simulink model "EOM_planar_vehicle_linmod"  (R2026a)
settings: Solver=VariableStepAuto  StopTime=10  MaxStep=deltaTMax
values from neighbouring files (symbols this model uses):
  CR = 0.75    [LineariseScript.m]    (also in PlanarVehicleScript.m)
  CT = 1/40    (= 0.025)    [LineariseScript.m]    (also in PlanarVehicleScript.m)
  Fmax = 10    [LineariseScript.m]    (also in PlanarVehicleScript.m)
  Ib = 0.5    [LineariseScript.m]    (also in PlanarVehicleScript.m)
  m = 10    [LineariseScript.m]    (also in PlanarVehicleScript.m)
  Mmax = 0.5    [LineariseScript.m]    (also in PlanarVehicleScript.m)
  u0 = [0.25 ... (first row only)    [LineariseScript.m]
  x0 = [10; -10; 0; 10; pi/2; 0]    [LineariseScript.m]    (also in PlanarVehicleScript.m = [10; -10; 0; 15; pi/2; 0])
settings Model: Creator=nuris  LastModifiedBy=nuris
settings DataIOCC: ExternalInput=getinputstruct(op_trim1)  InitialState=getstatestruct(op_trim1)

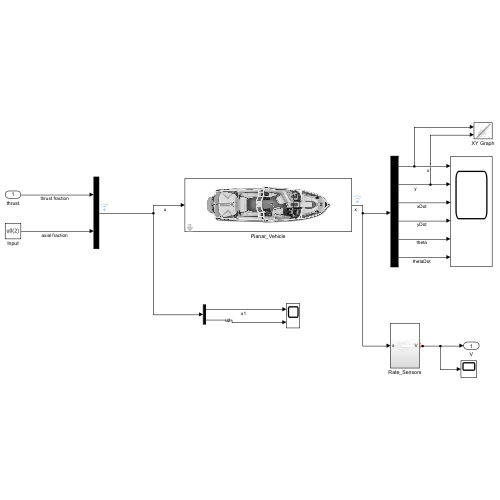
[thumbnail: Simulink's stored preview of the top-level diagram]
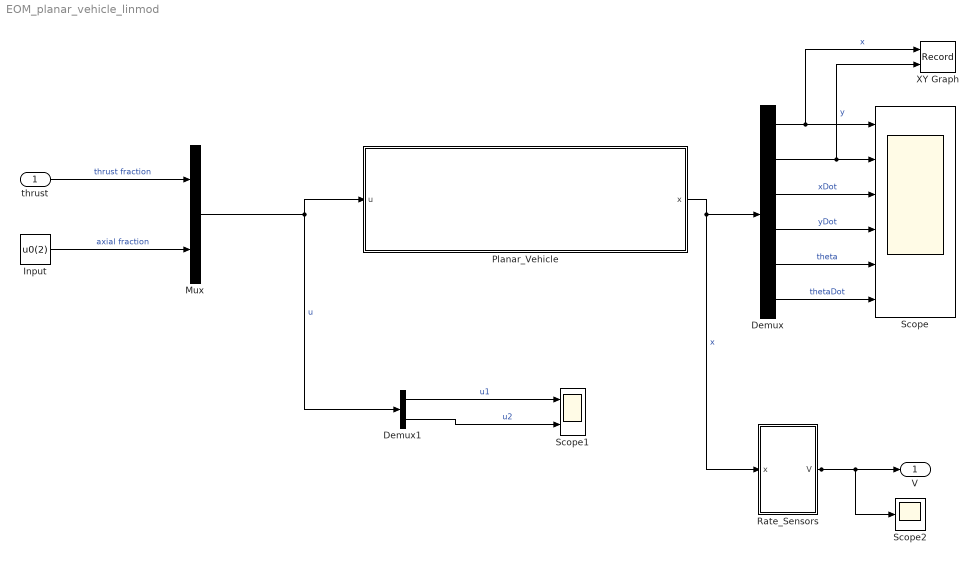
== system EOM_planar_vehicle_linmod ==
  thrust : Inport
  Demux : Demux  Outputs=6
  Demux1 : Demux  Outputs=2
  Input : Constant  Value=u0(2)
  Mux : Mux  Inputs=2
  Planar_Vehicle : Subsystem  mask(Subsystem (mask) (link)){x0=x0}
      mask prompts: x0 "Initial condition"
      mask help:
      | Represent a simple planar model.
      |
      | The state vector is
      |   x = [x;y;xdot;ydot;theta;thetadot]
      |
      | The control vector is
      |   u = [u1; u2]
      |
      | where:
      | u1 = fraction of axial thrust force in range [-1, 1] (-1 = full negative force, +1 = full positive force)
      | u2 = fraction of moment about CG in range [-1, 1] (-1 = full negative moment, +1 = full positive moment)
      |
      | INPUTS:
      |   u: 2x1 control vector
      |
      | OUTPUTS:
      |   x: 6x1 state vector
      mask Display: image(imread('C:\Users\nuris\Desktop\Michigan\Control\EOM_Planar_Vehicle\Boat.png'))
  Rate_Sensors : Subsystem
  Scope : Scope  NumInputPorts=6
      settings: ActiveDisplayYMinimum=-25.922686555926731  ActiveDisplayYMaximum=133.30417900334061
  Scope1 : Scope  NumInputPorts=2
      settings: ActiveDisplayYMinimum=-1  ActiveDisplayYMaximum=1
  Scope2 : Scope
      settings: ActiveDisplayYMinimum=14.999999999999581  ActiveDisplayYMaximum=15.000000000003784  DataLoggingVariableName=ScopeData2
  XY Graph : Record  NumPorts=2.0  FileSettingsInternal="{\"entries\":[{\"content\":{\"excelSettings\":{\"content\":{},\"type\":\"Streamout.ExcelSettings\"},\"parquetSettings\":{\"content\":{},\"type\":\"Streamout.ParquetSettings\"}},\"type\":\"Streamout.FileSettingStorage\",\"uuid\":\"\"}],\"packageUris\":[\"http:\\/\\/schema.mathworks.com\\/mf0\\/streamout_blocks\\/R2020a\"],\"version\":\"1.0\"}"  FrameSettings=[0, 0]  Layout=[1 1]  SignalsInternal="{\"entries\":[{\"content\":{\"signals\":[{\"content\":{\"blockPath\":[],\"dimensions\":[1],\"domain\":\"\",\"lineColor\":\"#edb120\",\"lineWidth\":2,\"port\":1,\"sid\":[\"\"],\"signalID\":1,\"signalName\":\"yDot\"},\"type\":\"RecordBlkView.Signal\",\"uuid\":\"\"},{\"content\":{\"blockPath\":[],\"dimensions\":[1],\"domain\":\"\",\"lineColor\":\"#7e2f8e\",\"lineWidth\":2,\"port\":1,\"sid\":[\"\"],\"signalID\":2},\"type\":\"RecordBlkView.Signal\",\"uuid\":\"\"},{\"content\":{\"blockPath\":[],\"dimensions\":[6],\"domain\":\"\",\"hasChildren\":true,\"lineColor\":\"#fe330a\",\"lineWidth\":2,\"port\":1,\"sid\":[\"\"],\"signalID\":3,\"signalName\":\"x\"},\"type\":\"RecordBlkView.Signal\",\"uuid\":\"\"},{\"content\":{\"blockPath\":[],\"channel\":[1],\"dimensions\":[6],\"domain\":\"\",\"lineColor\":\"#4dbeee\",\"lineWidth\":2,\"parentID\":3,\"port\":1,\"sid\":[\"\"],\"signalID\":4,\"signalName\":\"x\"},\"type\":\"RecordBlkView.Signal\",\"uuid\":\"\"},{\"content\":{\"blockPath\":[],\"dimensions\":[1],\"domain\":\"\",\"lineColor\":\"#a2142f\",\"plots\":[ 1 ],\"port\":1,\"sid\":[\"\"],\"signalID\":5,\"signalName\":\"x\"},\"type\":\"RecordBlkView.Signal\",\"uuid\":\"\"},{\"content\":{\"blockPath\":[],\"dimensions\":[1],\"domain\":\"\",\"lineColor\":\"#139fff\",\"plots\":[ 1 ],\"port\":2,\"sid\":[\"\"],\"signalID\":6,\"signalName\":\"y\"},\"type\":\"RecordBlkView.Signal\",\"uuid\":\"\"},{\"content\":{\"blockPath\":[],\"dimensions\":[2],\"domain\":\"\",\"hasChildren\":true,\"lineColor\":\"#edb120\",\"lineWidth\":2,\"port\":1,\"sid\":[\"\"],\"signalID\":7,\"signalName\":\"u\"},\"type\":\"RecordBlkView.Signal\",\"uuid\":\"\"},{\"content\":{\"blockPath\":[],\"channel\":[1],\"dimensions\":[2],\"domain\":\"\",\"lineColor\":\"#b746ff\",\"lineWidth\":2,\"parentID\":7,\"port\":1,\"sid\":[\"\"],\"signalID\":8,\"signalName\":\"u\"},\"type\":\"RecordBlkView.Signal\",\"uuid\":\"\"},{\"content\":{\"blockPath\":[],\"channel\":[2],\"dimensions\":[2],\"domain\":\"\",\"lineColor\":\"#77ac30\",\"lineWidth\":2,\"parentID\":7,\"port\":1,\"sid\":[\"\"],\"signalID\":9,\"signalName\":\"u\"},\"type\":\"RecordBlkView.Signal\",\"uuid\":\"\"}]},\"type\":\"RecordBlkView.InputSignals\",\"uuid\":\"\"}],\"packageUris\":[\"http:\\/\\/schema.mathworks.com\\/mf0\\/streamout_blocks\\/R2020a\"],\"version\":\"1.0\"}"  VisualizationBindings="{\"xyplotplugin\":{\"info\":[{\"series\":[{\"bindingParametersList\":[{\"parameter\":\"X-Axis\",\"signalID\":5,\"signalName\":\"x\"},{\"parameter\":\"Y-Axis\",\"signalID\":6,\"signalName\":\"y\"}],\"seriesID\":0}],\"subplotID\":1}]}}"  CompatibilityTag=XY
  V : Outport
  wires:
  Planar_Vehicle/1(x) -> Rate_Sensors/1(x), Demux/1  "x"
  Demux/1 -> XY Graph/1, Scope/1  "x"
  Demux/2 -> XY Graph/2, Scope/2  "y"
  Demux/3 -> Scope/3  "xDot"
  Demux/4 -> Scope/4  "yDot"
  Demux/5 -> Scope/5  "theta"
  Demux/6 -> Scope/6  "thetaDot"
  thrust/1 -> Mux/1  "thrust fraction"
  Input/1 -> Mux/2  "axial fraction"
  Mux/1 -> Demux1/1, Planar_Vehicle/1(u)  "u"
  Demux1/1 -> Scope1/1  "u1"
  Demux1/2 -> Scope1/2  "u2"
  Rate_Sensors/1(V) -> V/1, Scope2/1

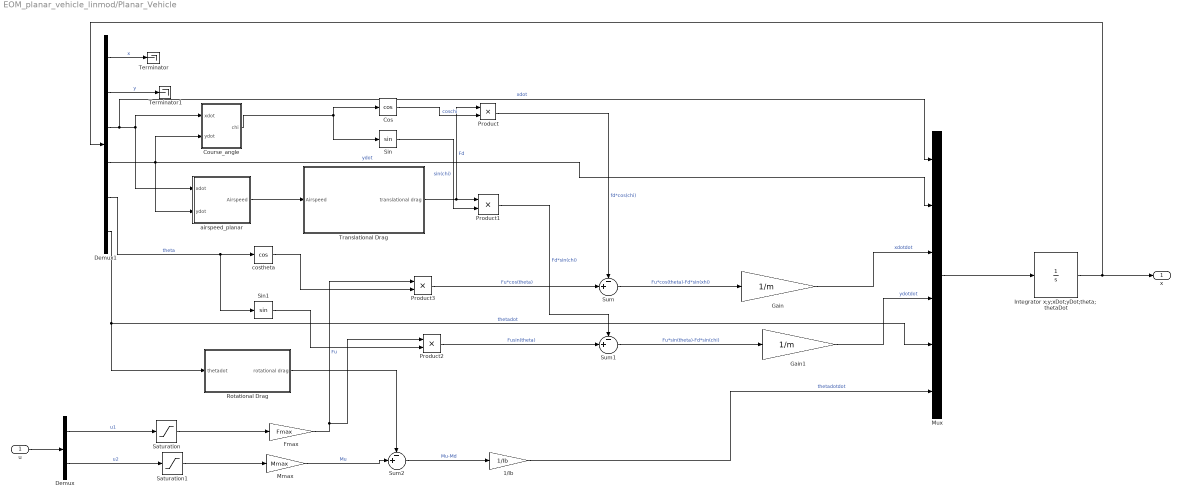
== system EOM_planar_vehicle_linmod/Planar_Vehicle ==
  u : Inport
  1/Ib : Gain  Gain=1/Ib
  Cos : Trigonometry  Operator=cos
  Course_angle : Subsystem
  Demux : Demux  Outputs=2
  Demux1 : Demux  Outputs=6
  Fmax : Gain  Gain=Fmax
  Gain : Gain  Gain=1/m
  Gain1 : Gain  Gain=1/m
  Integrator x;y;xDot;yDot;theta;thetaDot : Integrator  InitialCondition=x0
  Mmax : Gain  Gain=Mmax
  Mux : Mux  Inputs=6
  Product{,1..3} (4 alike) : Product
  Rotational Drag : Subsystem
  Saturation : Saturate  UpperLimit=1  LowerLimit=-1
  Saturation1 : Saturate  UpperLimit=1  LowerLimit=-1
  Sin : Trigonometry
  Sin1 : Trigonometry
  Sum : Sum  Inputs=-+|
  Sum1 : Sum  Inputs=-+|
  Sum2 : Sum  Inputs=-+|
  Terminator : Terminator
  Terminator1 : Terminator
  Translational Drag : Subsystem
  airspeed_planar : Subsystem
  costheta : Trigonometry  Operator=cos
  x : Outport
  wires:
  Demux/1 -> Saturation/1  "u1"
  Demux/2 -> Saturation1/1  "u2"
  Fmax/1 -> Product3/1, Product2/1  "Fu"
  Mmax/1 -> Sum2/2  "Mu"
  Demux1/1 -> Terminator/1  "x"
  Demux1/3 -> Mux/1, airspeed_planar/1(xdot), Course_angle/1(xdot)  "xdot"
  Demux1/4 -> airspeed_planar/2(ydot), Course_angle/2(ydot), Mux/2  "ydot"
  airspeed_planar/1(Airspeed) -> Translational Drag/1(Airspeed)
  Demux1/6 -> Mux/5, Rotational Drag/1(thetadot)  "thetadot"
  Demux1/2 -> Terminator1/1  "y"
  Course_angle/1(chi) -> Sin/1, Cos/1
  Product/1 -> Sum/1  "fd*cos(chi)"
  Translational Drag/1(translational drag) -> Product1/1, Product/1  "Fd"
  Cos/1 -> Product/2  "coschi"
  Sin/1 -> Product1/2  "sin(chi)"
  Product1/1 -> Sum1/1  "Fd*sin(chi)"
  Demux1/5 -> Sin1/1, costheta/1  "theta"
  Sin1/1 -> Product2/2
  Product2/1 -> Sum1/2  "Fusin(theta)"
  costheta/1 -> Product3/2
  Product3/1 -> Sum/2  "Fu*cos(theta)"
  Sum/1 -> Gain/1  "Fu*cos(theta)-Fd*sin(xhi)"
  Sum1/1 -> Gain1/1  "Fu*sin(theta)-Fd*sin(chi)"
  Gain/1 -> Mux/3  "xdotdot"
  Gain1/1 -> Mux/4  "ydotdot"
  Mux/1 -> Integrator x;y;xDot;yDot;theta;thetaDot/1
  Rotational Drag/1(rotational drag) -> Sum2/1
  Sum2/1 -> 1/Ib/1  "Mu-Md"
  1/Ib/1 -> Mux/6  "thetadotdot"
  Integrator x;y;xDot;yDot;theta;thetaDot/1 -> Demux1/1, x/1
  u/1 -> Demux/1
  Saturation/1 -> Fmax/1
  Saturation1/1 -> Mmax/1

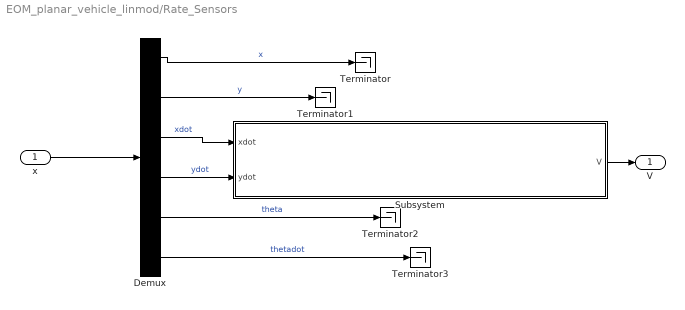
== system EOM_planar_vehicle_linmod/Rate_Sensors ==
  x : Inport
  Demux : Demux  Outputs=6
  Subsystem : Subsystem
  Terminator{,1..3} (4 alike) : Terminator
  V : Outport
  wires:
  x/1 -> Demux/1
  Demux/1 -> Terminator/1  "x"
  Demux/2 -> Terminator1/1  "y"
  Demux/6 -> Terminator3/1  "thetadot"
  Demux/4 -> Subsystem/2(ydot)  "ydot"
  Subsystem/1(V) -> V/1
  Demux/3 -> Subsystem/1(xdot)  "xdot"
  Demux/5 -> Terminator2/1  "theta"

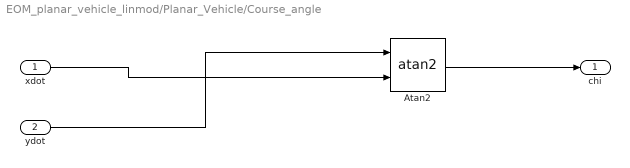
== system EOM_planar_vehicle_linmod/Planar_Vehicle/Course_angle ==
  xdot : Inport
  ydot : Inport  Port=2
  Atan2 : Trigonometry  Operator=atan2
  chi : Outport
  wires:
  ydot/1 -> Atan2/1
  Atan2/1 -> chi/1
  xdot/1 -> Atan2/2

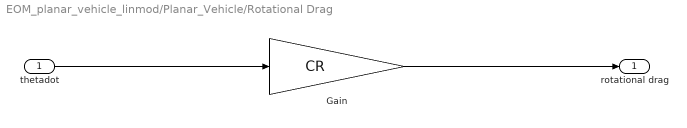
== system EOM_planar_vehicle_linmod/Planar_Vehicle/Rotational Drag ==
  thetadot : Inport
  Gain : Gain  Gain=CR
  rotational drag : Outport
  wires:
  Gain/1 -> rotational drag/1
  thetadot/1 -> Gain/1

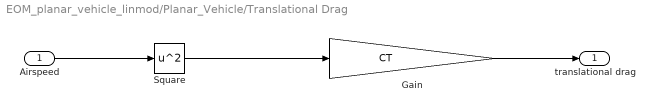
== system EOM_planar_vehicle_linmod/Planar_Vehicle/Translational Drag ==
  Airspeed : Inport
  Gain : Gain  Gain=CT
  Square : Math  Operator=square
  translational drag : Outport
  wires:
  Airspeed/1 -> Square/1
  Square/1 -> Gain/1
  Gain/1 -> translational drag/1

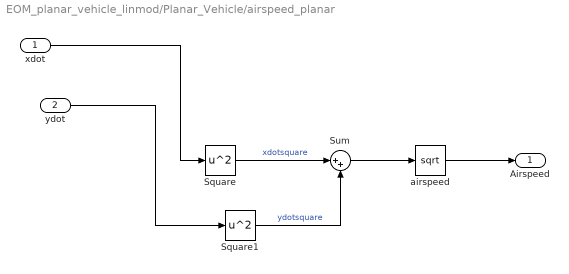
== system EOM_planar_vehicle_linmod/Planar_Vehicle/airspeed_planar ==
  xdot : Inport
  ydot : Inport  Port=2
  Square : Math  Operator=square
  Square1 : Math  Operator=square
  Sum : Sum  Inputs=|++
  airspeed : Sqrt
  Airspeed : Outport
  wires:
  ydot/1 -> Square1/1
  xdot/1 -> Square/1
  Square/1 -> Sum/1  "xdotsquare"
  Square1/1 -> Sum/2  "ydotsquare"
  Sum/1 -> airspeed/1
  airspeed/1 -> Airspeed/1

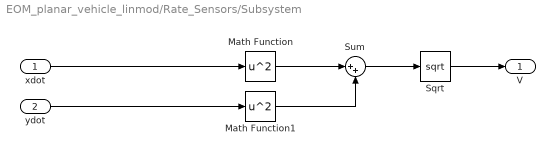
== system EOM_planar_vehicle_linmod/Rate_Sensors/Subsystem ==
  xdot : Inport
  ydot : Inport  Port=2
  Math Function : Math  Operator=square
  Math Function1 : Math  Operator=square
  Sqrt : Sqrt
  Sum : Sum  Inputs=|++
  V : Outport
  wires:
  Sum/1 -> Sqrt/1
  Sqrt/1 -> V/1
  Math Function1/1 -> Sum/2
  Math Function/1 -> Sum/1
  ydot/1 -> Math Function1/1
  xdot/1 -> Math Function/1
